simulink model "external_memory_test"  (R2020b)
settings: Solver=FixedStepDiscrete  StartTime=0.0  StopTime=80  RelTol=1e-3
InitFcn:
  | Feature_Width = 64;
  | Feature_Height = 64;
  | Weight_Width = 3;
  | Weight_Height = 3;
  | external_memory_test_init;
values from neighbouring files (symbols this model uses):
  Burst_Length = Feature_Weight_Length    [external_memory_test_init.m]
  byPass = 1    [external_memory_test_init.m]
  Conv_Padding = 0    [external_memory_test_init.m]
  Conv_Stride = 1    [external_memory_test_init.m]
  DDR_Depth = Weight_Length + Feature_Length + outFeature_Length    [external_memory_test_init.m]
  ddrInitData = single((rand(1,DDR_Depth)))    [external_memory_test_init.m]
  Duty_Cycle = 0.5    [external_memory_test_init.m]
  Feature_Area = Feature_Width * Feature_Height    [external_memory_test_init.m]
  Feature_Length = Phase_In * Feature_Area    [external_memory_test_init.m]
  inChannel = 3    [external_memory_test_init.m]
  outChannel = 2    [external_memory_test_init.m]
  outFeature_Length = outFeature_Width * outFeature_Height * Phase_Out    [external_memory_test_init.m]
  Pool_Stride = 2    [external_memory_test_init.m]
  Pool_Width = 2    [external_memory_test_init.m]
  Tc = 1    [external_memory_test_init.m]
  Ti = 1    [external_memory_test_init.m]
  To = 1    [external_memory_test_init.m]
  Tr = 1    [external_memory_test_init.m]
  Weight_Length = Phase_In * Weight_Area * Phase_Out    [external_memory_test_init.m]
undefined symbols (not defined in the file or in its folder): Conv_Step, Pool_Step, sigbuilder_block
libraries: hdlsllib x85, simulink x44, visionhdlutilities x16
(part 4 of 6)

== system external_memory_test/DUT/2DConvPE V1.3/Window Selector ==
  In1 : Inport
  valid : Inport  Port=2
  step : Inport  Port=3
  Add : Sum  Inputs=+-
  Compare To Zero : simulink/Logic and Bit Operations/Compare To Zero  relop===  OutDataTypeStr=boolean
  Constant : Constant  OutDataTypeStr=uint32
  Delay : Delay
  Delay1 : Delay  DelayLength=3
  Delay2 : Delay  DelayLength=1
  Delay3 : Delay  DelayLength=1
  Delay4 : Delay  DelayLength=1
  Logical Operator : Logic  Operator=NOT  AllPortsSameDT=off  OutDataTypeStr=boolean
  Logical Operator1 : Logic  Operator=OR  AllPortsSameDT=off  OutDataTypeStr=boolean
  Logical Operator2 : Logic  AllPortsSameDT=off  OutDataTypeStr=boolean
  Relational Operator : RelationalOperator  OutDataTypeStr=boolean  RndMeth=Nearest
  Selector1 : Selector  InputPortWidth=3  IndexOptions=Index vector (dialog)  Indices=[1]  OutputSizes=1
  Selector2 : Selector  InputPortWidth=3  IndexOptions=Index vector (dialog)  Indices=[2]  OutputSizes=1
  Selector3 : Selector  InputPortWidth=3  IndexOptions=Index vector (dialog)  Indices=[3]  OutputSizes=1
  Selector4 : Selector  InputPortWidth=3  IndexOptions=Index vector (dialog)  Indices=[1]  OutputSizes=1
  Selector5 : Selector  InputPortWidth=3  IndexOptions=Index vector (dialog)  Indices=[2]  OutputSizes=1
  Selector6 : Selector  InputPortWidth=3  IndexOptions=Index vector (dialog)  Indices=[3]  OutputSizes=1
  Selector7 : Selector  InputPortWidth=3  IndexOptions=Index vector (dialog)  Indices=[1]  OutputSizes=1
  Selector8 : Selector  InputPortWidth=3  IndexOptions=Index vector (dialog)  Indices=[2]  OutputSizes=1
  Selector9 : Selector  InputPortWidth=3  IndexOptions=Index vector (dialog)  Indices=[3]  OutputSizes=1
  Step Counter : hdlsllib/Sources/HDL Counter  CountType=Free running  CountInit=0  CountStep=1  CountMax=2^15  CountFromType=Initial value  CountFrom=0  CountResetPort=on  CountLoadPort=off  CountEnbPort=on  CountDirPort=off  CountDataType=Unsigned  CountWordLen=32  CountFracLen=0  CountSampTime=1
  Out1 : Outport
  Out2 : Outport  Port=2
  Out3 : Outport  Port=3
  Out4 : Outport  Port=4
  Out5 : Outport  Port=5
  Out6 : Outport  Port=6
  Out7 : Outport  Port=7
  Out8 : Outport  Port=8
  Out9 : Outport  Port=9
  Valid : Outport  Port=10
  wires:
  Selector2/1 -> Out2/1
  In1/1 -> Delay2/1, Delay1/1, Delay/1
  Selector1/1 -> Out1/1
  Selector3/1 -> Out3/1
  Selector8/1 -> Out5/1
  Selector9/1 -> Out6/1
  Selector7/1 -> Out4/1
  Delay/1 -> Selector9/1, Selector8/1, Selector7/1
  Selector5/1 -> Out8/1
  Selector6/1 -> Out9/1
  Selector4/1 -> Out7/1
  Delay1/1 -> Selector6/1, Selector5/1, Selector4/1
  Relational Operator/1 -> Logical Operator1/1
  Constant/1 -> Add/2
  Logical Operator2/1 -> Valid/1
  Compare To Zero/1 -> Logical Operator2/1
  Logical Operator1/1 -> Step Counter/1
  Logical Operator/1 -> Logical Operator1/2
  Delay4/1 -> Add/1
  Step Counter/1 -> Compare To Zero/1, Relational Operator/1
  Delay3/1 -> Logical Operator2/2, Step Counter/2, Logical Operator/1
  Add/1 -> Relational Operator/2
  Delay2/1 -> Selector3/1, Selector2/1, Selector1/1
  valid/1 -> Delay3/1
  step/1 -> Delay4/1

== system external_memory_test/DUT/DDR_Access/EdgeDetection2 ==
  In1 : Inport
  Delay : Delay  DelayLength=1
  Logical Operator : Logic  AllPortsSameDT=off  OutDataTypeStr=boolean
  Logical Operator1 : Logic  Operator=NOT  AllPortsSameDT=off  OutDataTypeStr=boolean
  Out1 : Outport  VectorParamsAs1DForOutWhenUnconnected=off
  wires:
  In1/1 -> Logical Operator/2, Delay/1
  Delay/1 -> Logical Operator1/1
  Logical Operator1/1 -> Logical Operator/1
  Logical Operator/1 -> Out1/1

== system external_memory_test/DUT/Input Buffer/Feature Buffer ==
  ram_wr_data : Inport
  ram_wr_addr : Inport  Port=2
  ram_wr_en : Inport  Port=3
  ram_rd_addr : Inport  Port=4
  Data Type Conversion : DataTypeConversion  OutDataTypeStr=uint16
  Data Type Conversion1 : DataTypeConversion  OutDataTypeStr=uint16
  Simple Dual Port RAM System : hdlsllib/HDL RAMs/Simple Dual Port RAM System  RAMType=Simple dual port  WriteOutputValue=New data  RAMInitialValue=0  SimulateUsing=Code generation
      settings: SourceProductName=HDL Coder
  ram_rd_data : Outport  VectorParamsAs1DForOutWhenUnconnected=off
  wires:
  Data Type Conversion/1 -> Simple Dual Port RAM System/2
  Data Type Conversion1/1 -> Simple Dual Port RAM System/4
  ram_wr_addr/1 -> Data Type Conversion/1
  Simple Dual Port RAM System/1 -> ram_rd_data/1
  ram_rd_addr/1 -> Data Type Conversion1/1
  ram_wr_en/1 -> Simple Dual Port RAM System/3
  ram_wr_data/1 -> Simple Dual Port RAM System/1

== system external_memory_test/DUT/Input Buffer/OutAddressLogic ==
  Weight_Length : Inport
  Weight_Area : Inport  Port=2
  Feature_Length : Inport  Port=3
  Feature_Area : Inport  Port=4
  Feature_Width : Inport  Port=5
  Feature_Height : Inport  Port=6
  outChannel : Inport  Port=7
  Out_enable : Inport  Port=8
  FeatureAddressOut : Subsystem
  Subsystem : Subsystem
  weight_ram_rd_addr : Outport
  featture_ram_rd_addr : Outport  Port=2
  feature_data_valid : Outport  Port=3
  weight_data_valid : Outport  Port=4
  PhaseOut_Count : Outport  Port=5
  wires:
  Feature_Length/1 -> FeatureAddressOut/1(Feature_Length)
  Out_enable/1 -> FeatureAddressOut/2(Out_Enable)
  Feature_Width/1 -> FeatureAddressOut/3(Feature_Width)
  FeatureAddressOut/1(count) -> featture_ram_rd_addr/1
  FeatureAddressOut/2(Out2) -> Subsystem/1(In1), feature_data_valid/1
  outChannel/1 -> FeatureAddressOut/4(outChannel)
  Feature_Area/1 -> Subsystem/2(Feature_Area)
  Weight_Length/1 -> Subsystem/3(Weight_Length)
  Weight_Area/1 -> Subsystem/4(Weight_Area)
  Subsystem/1(weight_ram_rd_addr) -> weight_ram_rd_addr/1
  Subsystem/2(valid) -> weight_data_valid/1
  Feature_Height/1 -> FeatureAddressOut/5(Feature_Height)
  FeatureAddressOut/3(PhaseOut_Count) -> PhaseOut_Count/1

== system external_memory_test/DUT/Input Buffer/SeparateWrite ==
  In1 : Inport
  In2 : Inport  Port=2
  Weight_Length : Inport  Port=3
  Compare To Zero : simulink/Logic and Bit Operations/Compare To Zero  relop=<  OutDataTypeStr=boolean
  Data Type Conversion : DataTypeConversion
  Logical Operator : Logic  Operator=NOT  AllPortsSameDT=off  OutDataTypeStr=boolean
  Logical Operator1 : Logic  AllPortsSameDT=off  OutDataTypeStr=boolean
  Logical Operator2 : Logic  AllPortsSameDT=off  OutDataTypeStr=boolean
  Minus : Sum  Inputs=+-
  Out1 : Outport
  Out2 : Outport  Port=2
  Out3 : Outport  Port=3
  wires:
  Logical Operator/1 -> Logical Operator2/2
  Minus/1 -> Data Type Conversion/1, Compare To Zero/1
  Logical Operator2/1 -> Out3/1
  Compare To Zero/1 -> Logical Operator/1, Logical Operator1/2
  In1/1 -> Logical Operator2/1, Logical Operator1/1
  In2/1 -> Minus/1
  Logical Operator1/1 -> Out1/1
  Weight_Length/1 -> Minus/2
  Data Type Conversion/1 -> Out2/1

== system external_memory_test/DUT/Input Buffer/Subsystem1 ==
  In1 : Inport
  Subsystem : Subsystem
  Terminator{,1..7} (8 alike) : Terminator
  Weight_Length : Outport
  Weight_Area : Outport  Port=2
  Feature_Length : Outport  Port=3
  Feature_Area : Outport  Port=4
  Feature_Width : Outport  Port=5
  Feature_Height : Outport  Port=6
  outChannel : Outport  Port=7
  wires:
  Subsystem/2(Weight_Area) -> Weight_Area/1
  Subsystem/12(outFeature_Height) -> Terminator5/1
  Subsystem/10(outFeature_Area) -> Terminator3/1
  Subsystem/13(Conv_Step) -> Terminator7/1
  Subsystem/9(outFeature_Length) -> Terminator2/1
  Subsystem/4(Weight_Height) -> Terminator1/1
  Subsystem/14(inChannel) -> Terminator6/1
  Subsystem/11(outFeature_Width) -> Terminator4/1
  Subsystem/3(Weight_Width) -> Terminator/1
  Subsystem/8(Feature_Height) -> Feature_Height/1
  Subsystem/1(Weight_Length) -> Weight_Length/1
  In1/1 -> Subsystem/1(In1)
  Subsystem/15(outChannel) -> outChannel/1
  Subsystem/5(Feature_Length) -> Feature_Length/1
  Subsystem/6(Feature_Area) -> Feature_Area/1
  Subsystem/7(Feature_Width) -> Feature_Width/1

== system external_memory_test/DUT/Input Buffer/Weight Buffer ==
  ram_wr_data : Inport
  ram_wr_addr : Inport  Port=2
  ram_wr_en : Inport  Port=3
  ram_rd_addr : Inport  Port=4
  Data Type Conversion : DataTypeConversion  OutDataTypeStr=uint16
  Data Type Conversion1 : DataTypeConversion  OutDataTypeStr=uint16
  Simple Dual Port RAM System : hdlsllib/HDL RAMs/Simple Dual Port RAM System  RAMType=Simple dual port  WriteOutputValue=New data  RAMInitialValue=0  SimulateUsing=Code generation
      settings: SourceProductName=HDL Coder
  ram_rd_data : Outport  VectorParamsAs1DForOutWhenUnconnected=off
  wires:
  Data Type Conversion/1 -> Simple Dual Port RAM System/2
  Data Type Conversion1/1 -> Simple Dual Port RAM System/4
  ram_wr_addr/1 -> Data Type Conversion/1
  Simple Dual Port RAM System/1 -> ram_rd_data/1
  ram_rd_addr/1 -> Data Type Conversion1/1
  ram_wr_en/1 -> Simple Dual Port RAM System/3
  ram_wr_data/1 -> Simple Dual Port RAM System/1

== system external_memory_test/DUT/outBuffer/Out Buffer ==
  ram_wr_data : Inport
  ram_wr_addr : Inport  Port=2
  ram_wr_en : Inport  Port=3
  ram_rd_addr : Inport  Port=4
  Cast : DataTypeConversion  OutDataTypeStr=uint32
  Data Type Conversion : DataTypeConversion  OutDataTypeStr=uint16
  Data Type Conversion1 : DataTypeConversion  OutDataTypeStr=uint16
  Simple Dual Port RAM System : hdlsllib/HDL RAMs/Simple Dual Port RAM System  RAMType=Simple dual port  WriteOutputValue=New data  RAMInitialValue=0  SimulateUsing=Code generation
      settings: SourceProductName=HDL Coder
  ram_rd_data : Outport  VectorParamsAs1DForOutWhenUnconnected=off
  wires:
  Data Type Conversion/1 -> Simple Dual Port RAM System/2
  Data Type Conversion1/1 -> Simple Dual Port RAM System/4
  ram_wr_addr/1 -> Data Type Conversion/1
  Simple Dual Port RAM System/1 -> Cast/1
  ram_rd_addr/1 -> Data Type Conversion1/1
  ram_wr_en/1 -> Simple Dual Port RAM System/3
  ram_wr_data/1 -> Simple Dual Port RAM System/1
  Cast/1 -> ram_rd_data/1

== system external_memory_test/InputSubsystem/Subsystem1/Signal Builder-Simulation ==
  Demux : Demux  Tag=STV Demux  Outputs=3
      settings: DisplayOption=none
  FromWs : FromWorkspace  Tag=STV FromWs  VariableName=tuvar  SampleTime=0.001  ZeroCross=off  OutputAfterFinalValue=Holding final value
      SigBuilderData=|
      | common.afterFinalStr = 'Hold final value'
      | common.sampleTime = '0.001'
      | dataSet.timeRange = [0 80]
      | dataSet.name = 'Group 1'
      | sbobj.Groups.Name = 'Group 1'
      | sbobj.Groups.Signals(1).Name = 'start'
      | sbobj.Groups.Signals(1).XData = [0 29 29 30 30 60 60 61 61 80]
      | sbobj.Groups.Signals(1).YData = [0 0 1 1 0 0 1 1 0 0]
      | sbobj.Groups.Signals(2).Name = 'from_ddr_to_ram'
      | sbobj.Groups.Signals(2).XData = [0 58.6 58.6 80]
      | sbobj.Groups.Signals(2).YData = [1 1 0 0]
      | sbobj.Groups.Signals(3).Name = 'conv_en'
      | sbobj.Groups.Signals(3).XData = [0 31.3 31.3 50 80]
      | sbobj.Groups.Signals(3).YData = [0 0 1 0.99 0.99]
      | sbobj.Groups.TimeRange = [0 80]
  start : Outport  Tag=STV Outport  VectorParamsAs1DForOutWhenUnconnected=off
  from_ddr_to_ram : Outport  Tag=STV Outport  Port=2  VectorParamsAs1DForOutWhenUnconnected=off
  conv_en : Outport  Tag=STV Outport  Port=3
  wires:
  Demux/1 -> start/1
  Demux/2 -> from_ddr_to_ram/1
  Demux/3 -> conv_en/1
  FromWs/1 -> Demux/1

== system external_memory_test/OutputSubsystem/to_MATLAB/to Matlab ==
  In1 : Inport
  Enable : EnablePort
  To Workspace : ToWorkspace  VariableName=DDR_WR_DATA  SampleTime=-1
  wires:
  In1/1 -> To Workspace/1

== system external_memory_test/DDR/wrLogic/Wr_control/AckGen ==
  axiWrLen : Inport
  wrEnb : Inport  Port=2
  ddr_wr_rdy : Inport  Port=3
  Delay : Delay  DelayLength=1
  Delay1 : Delay  DelayLength=1
  ValwrLenCnt : hdlsllib/Sources/HDL Counter  CountType=Free running  CountInit=0  CountStep=1  CountMax=DDR3_DEPTH  CountFromType=Initial value  CountFrom=0  CountResetPort=on  CountLoadPort=off  CountEnbPort=on  CountDirPort=off  CountDataType=Unsigned  CountWordLen=32  CountFracLen=0  CountSampTime=1
  axiWrLen!=0 : simulink/Logic and Bit Operations/Compare To Constant  relop=~=  const=0  OutDataTypeStr=boolean
  "axiWrLen-1==cnt & axiWrLen!=0 " : Logic  Inputs=3  IconShape=distinctive  AllPortsSameDT=off  OutDataTypeStr=boolean
  axiWrLen==cnt+1 : RelationalOperator  Operator===  OutDataTypeStr=boolean  RndMeth=Nearest
  edgeDet : Subsystem
  if cnt < axiWrLen : RelationalOperator  Operator=<=  OutDataTypeStr=boolean  RndMeth=Nearest
  ram_wr_enb cond : Logic  IconShape=distinctive  AllPortsSameDT=off  OutDataTypeStr=boolean
  ram_wr_enb cond1 : Logic  IconShape=distinctive  AllPortsSameDT=off  OutDataTypeStr=boolean
  ack : Outport  VectorParamsAs1DForOutWhenUnconnected=off
  ValAddEnb : Outport  Port=2  VectorParamsAs1DForOutWhenUnconnected=off
  ram_addr : Outport  Port=3  VectorParamsAs1DForOutWhenUnconnected=off
  wires:
  "axiWrLen-1==cnt & axiWrLen!=0 "/1 -> edgeDet/1(ackIn)
  edgeDet/1(ackOut) -> ack/1, Delay/1
  axiWrLen==cnt+1/1 -> "axiWrLen-1==cnt & axiWrLen!=0 "/2
  axiWrLen!=0/1 -> "axiWrLen-1==cnt & axiWrLen!=0 "/3
  wrEnb/1 -> ram_wr_enb cond/1
  if cnt < axiWrLen/1 -> ram_wr_enb cond1/2
  axiWrLen/1 -> axiWrLen==cnt+1/2, axiWrLen!=0/1, if cnt < axiWrLen/2
  ValwrLenCnt/1 -> axiWrLen==cnt+1/1, if cnt < axiWrLen/1, ram_addr/1
  ddr_wr_rdy/1 -> ram_wr_enb cond/2
  ram_wr_enb cond/1 -> ram_wr_enb cond1/1, Delay1/1, ValwrLenCnt/2
  ram_wr_enb cond1/1 -> ValAddEnb/1
  Delay/1 -> ValwrLenCnt/1
  Delay1/1 -> "axiWrLen-1==cnt & axiWrLen!=0 "/1

== system external_memory_test/DUT/2DConvPE V1.0/Address Logic/  ==
  In1 : Inport
  In2 : Inport  Port=2
  Constant1 : Constant  Value=0  OutDataTypeStr=uint32
  Constant2 : Constant  Value=0  OutDataTypeStr=uint32
  Logical Operator3 : Logic  Operator=NOT  AllPortsSameDT=off  OutDataTypeStr=boolean
  Switch : Switch  Criteria=u2 ~= 0
  Switch1 : Switch  Criteria=u2 ~= 0
  addr_bit_sel1 : hdlsllib/Logic and Bit Operations/Bit Slice  lidx=12  ridx=0
  addr_bit_sel2 : hdlsllib/Logic and Bit Operations/Bit Slice  lidx=12  ridx=0
  W : Outport
  R : Outport  Port=2
  wires:
  In2/1 -> Switch/2, Logical Operator3/1
  Constant1/1 -> Switch/1
  Switch1/1 -> addr_bit_sel1/1
  In1/1 -> Switch1/3, Switch/3
  Logical Operator3/1 -> Switch1/2
  Constant2/1 -> Switch1/1
  Switch/1 -> addr_bit_sel2/1
  addr_bit_sel1/1 -> W/1  "vec_wr_addr"
  addr_bit_sel2/1 -> R/1  "vec_wr_addr"

== system external_memory_test/DUT/2DConvPE V1.0/LIne Buffer/Line Buffer ==
  Stream_In : Inport
  Stream_Valid : Inport  Port=2
  Feature_Area : Inport  Port=3
  Feature_Width : Inport  Port=4
  CtrlGen : Subsystem
  Line Buffer : visionhdlutilities/Line Buffer  NeighborhoodSize=[3 1]  PaddingMethod=Constant  PaddingValue=0  LineBufferSize=128  SimulateUsing=Code generation
      settings: SourceProductBaseCode=VT
  pixel : Outport
  ctrl : Outport  Port=2
  shftEnable : Outport  Port=3
  wires:
  Feature_Area/1 -> CtrlGen/3(Feature_Area)
  Line Buffer/2 -> ctrl/1
  CtrlGen/1(StreamOut) -> Line Buffer/1
  Feature_Width/1 -> CtrlGen/4(Feature_Width)
  Stream_In/1 -> CtrlGen/1(Stream_In)
  CtrlGen/2(Ctrl) -> Line Buffer/2
  Stream_Valid/1 -> CtrlGen/2(Stream_Valid)
  Line Buffer/3 -> shftEnable/1
  Line Buffer/1 -> pixel/1

== system external_memory_test/DUT/2DConvPE V1.0/LIne Buffer/OutValidGen ==
  In1 : Inport
  Weight_Width : Inport  Port=2
  Feature_Height : Inport  Port=3
  Compare To Constant : simulink/Logic and Bit Operations/Compare To Constant  relop=>  const=0  OutDataTypeStr=boolean
  Constant : Constant  OutDataTypeStr=uint32  SampleTime=-1
  Delay2 : Delay  DelayLength=1
  Logical Operator1 : Logic  Operator=NOT  AllPortsSameDT=off  OutDataTypeStr=boolean
  Logical Operator2 : Logic  Operator=OR  AllPortsSameDT=off  OutDataTypeStr=boolean
  Logical Operator3 : Logic  Inputs=4  AllPortsSameDT=off  OutDataTypeStr=boolean
  Logical Operator4 : Logic  Operator=NOT  AllPortsSameDT=off  OutDataTypeStr=boolean
  Logical Operator5 : Logic  Operator=OR  AllPortsSameDT=off  OutDataTypeStr=boolean
  Logical Operator6 : Logic  Operator=NOT  Inputs=3  AllPortsSameDT=off  OutDataTypeStr=boolean
  Minus1 : Sum  Inputs=+--
  Minus2 : Sum  Inputs=+-
  NumRow_Counter : hdlsllib/Sources/HDL Counter  CountType=Free running  CountInit=0  CountStep=1  CountMax=2^15  CountFromType=Initial value  CountFrom=0  CountResetPort=on  CountLoadPort=off  CountEnbPort=on  CountDirPort=off  CountDataType=Unsigned  CountWordLen=32  CountFracLen=0  CountSampTime=1
  Pixel Control Bus Selector : BusSelector  OutputSignals=hStart,hEnd,vStart,vEnd,valid
  Relational Operator1 : RelationalOperator  Operator=<  OutDataTypeStr=boolean  RndMeth=Nearest
  Relational Operator2 : RelationalOperator  Operator=<=  OutDataTypeStr=boolean  RndMeth=Nearest
  Row_Counter : hdlsllib/Sources/HDL Counter  CountType=Free running  CountInit=0  CountStep=1  CountMax=2^15  CountFromType=Initial value  CountFrom=0  CountResetPort=on  CountLoadPort=off  CountEnbPort=on  CountDirPort=off  CountDataType=Unsigned  CountWordLen=32  CountFracLen=0  CountSampTime=1
  Terminator1 : Terminator
  valid : Outport
  wires:
  Compare To Constant/1 -> Logical Operator3/2
  NumRow_Counter/1 -> Relational Operator2/2, Compare To Constant/1
  Pixel Control Bus Selector/1 -> NumRow_Counter/2, Logical Operator2/1  "<hStart>"
  Minus2/1 -> Relational Operator2/1
  Relational Operator1/1 -> Logical Operator4/1
  Logical Operator1/1 -> Logical Operator2/2
  Pixel Control Bus Selector/3 -> Logical Operator5/1  "<vStart>"
  Feature_Height/1 -> Minus2/1
  Minus1/1 -> Relational Operator1/2
  Row_Counter/1 -> Relational Operator1/1
  Pixel Control Bus Selector/5 -> Logical Operator1/1, Row_Counter/2, Logical Operator3/3  "<valid>"
  Weight_Width/1 -> Minus1/1
  Pixel Control Bus Selector/2 -> Terminator1/1  "<hEnd>"
  Delay2/1 -> Pixel Control Bus Selector/1
  Constant/1 -> Minus1/3, Minus1/2, Minus2/2
  Logical Operator6/1 -> Logical Operator3/1
  Logical Operator5/1 -> NumRow_Counter/1
  Pixel Control Bus Selector/4 -> Logical Operator5/2  "<vEnd>"
  Relational Operator2/1 -> Logical Operator6/1
  Logical Operator2/1 -> Row_Counter/1
  Logical Operator4/1 -> Logical Operator3/4
  Logical Operator3/1 -> valid/1
  In1/1 -> Delay2/1

== system external_memory_test/DUT/2DConvPE V1.0/MaxPooling/Comparator ==
  In1 : Inport
  In2 : Inport  Port=2
  In3 : Inport  Port=3
  In4 : Inport  Port=4
  Valid : Inport  Port=5
  Delay{,1..4} (5 alike) : Delay  DelayLength=1
  Relational Operator : RelationalOperator  Operator=>  OutDataTypeStr=boolean  RndMeth=Nearest
  Relational Operator1 : RelationalOperator  Operator=>  OutDataTypeStr=boolean  RndMeth=Nearest
  Relational Operator2 : RelationalOperator  Operator=>  OutDataTypeStr=boolean  RndMeth=Nearest
  Switch : Switch  Criteria=u2 > Threshold
  Switch1 : Switch  Criteria=u2 > Threshold
  Switch2 : Switch  Criteria=u2 > Threshold
  Out1 : Outport
  outvalid : Outport  Port=2
  wires:
  Switch1/1 -> Relational Operator2/2, Switch2/3
  Switch/1 -> Switch2/1, Relational Operator2/1
  Delay/1 -> Switch/1, Relational Operator/1
  Relational Operator/1 -> Switch/2
  Relational Operator1/1 -> Switch1/2
  In2/1 -> Delay1/1
  In3/1 -> Delay2/1
  Relational Operator2/1 -> Switch2/2
  In4/1 -> Delay3/1
  Switch2/1 -> Out1/1
  Valid/1 -> Delay4/1
  Delay1/1 -> Relational Operator/2, Switch/3
  Delay2/1 -> Switch1/1, Relational Operator1/1
  In1/1 -> Delay/1
  Delay3/1 -> Relational Operator1/2, Switch1/3
  Delay4/1 -> outvalid/1

== system external_memory_test/DUT/2DConvPE V1.0/MaxPooling/Line Buffer1 ==
  Stream_In : Inport
  Stream_Valid : Inport  Port=2
  Feature_Area : Inport  Port=3
  Feature_Width : Inport  Port=4
  CtrlGen : Subsystem
  Line Buffer : visionhdlutilities/Line Buffer  NeighborhoodSize=[2 1]  PaddingMethod=Constant  PaddingValue=0  LineBufferSize=128  SimulateUsing=Code generation
      settings: SourceProductBaseCode=VT
  pixel : Outport
  ctrl : Outport  Port=2
  shftEnable : Outport  Port=3
  wires:
  Feature_Area/1 -> CtrlGen/3(Feature_Area)
  Line Buffer/2 -> ctrl/1
  CtrlGen/1(StreamOut) -> Line Buffer/1
  Feature_Width/1 -> CtrlGen/4(Feature_Width)
  Stream_In/1 -> CtrlGen/1(Stream_In)
  CtrlGen/2(Ctrl) -> Line Buffer/2
  Stream_Valid/1 -> CtrlGen/2(Stream_Valid)
  Line Buffer/3 -> shftEnable/1
  Line Buffer/1 -> pixel/1

== system external_memory_test/DUT/2DConvPE V1.0/MaxPooling/OutValidGen ==
  ctrl : Inport
  Window_Width : Inport  Port=2
  Feature_Height : Inport  Port=3
  Compare To Constant : simulink/Logic and Bit Operations/Compare To Constant  Commented=on  relop=>  const=0  OutDataTypeStr=boolean
  Constant : Constant  OutDataTypeStr=uint32  SampleTime=-1
  Delay36 : Delay  DelayLength=1
  Logical Operator1 : Logic  Operator=NOT  AllPortsSameDT=off  OutDataTypeStr=boolean
  Logical Operator3 : Logic  Inputs=3  AllPortsSameDT=off  OutDataTypeStr=boolean
  Logical Operator4 : Logic  Operator=NOT  AllPortsSameDT=off  OutDataTypeStr=boolean
  Logical Operator5 : Logic  Operator=OR  AllPortsSameDT=off  OutDataTypeStr=boolean
  Logical Operator6 : Logic  Operator=NOT  Inputs=3  AllPortsSameDT=off  OutDataTypeStr=boolean
  Minus1 : Sum  Inputs=+-
  Minus2 : Sum  Inputs=+-
  NumRow_Counter : hdlsllib/Sources/HDL Counter  CountType=Free running  CountInit=0  CountStep=1  CountMax=2^15  CountFromType=Initial value  CountFrom=0  CountResetPort=on  CountLoadPort=off  CountEnbPort=on  CountDirPort=off  CountDataType=Unsigned  CountWordLen=32  CountFracLen=0  CountSampTime=1
  Pixel Control Bus Selector : BusSelector  OutputSignals=hStart,hEnd,vStart,vEnd,valid
  Relational Operator1 : RelationalOperator  Operator=<  OutDataTypeStr=boolean  RndMeth=Nearest
  Relational Operator2 : RelationalOperator  Operator=<=  OutDataTypeStr=boolean  RndMeth=Nearest
  Row_Counter : hdlsllib/Sources/HDL Counter  CountType=Free running  CountInit=0  CountStep=1  CountMax=2^15  CountFromType=Initial value  CountFrom=0  CountResetPort=on  CountLoadPort=off  CountEnbPort=on  CountDirPort=off  CountDataType=Unsigned  CountWordLen=32  CountFracLen=0  CountSampTime=1
  Terminator1 : Terminator
  Out1 : Outport
  wires:
  Compare To Constant/1 -> ?
  NumRow_Counter/1 -> Relational Operator2/2, Compare To Constant/1
  Pixel Control Bus Selector/1 -> NumRow_Counter/2  "<hStart>"
  Minus2/1 -> Relational Operator2/1
  Relational Operator1/1 -> Logical Operator4/1
  Pixel Control Bus Selector/3 -> Logical Operator5/1  "<vStart>"
  Feature_Height/1 -> Minus2/1
  Minus1/1 -> Relational Operator1/2
  Row_Counter/1 -> Relational Operator1/1
  Pixel Control Bus Selector/5 -> Row_Counter/2, Logical Operator1/1, Logical Operator3/2  "<valid>"
  Window_Width/1 -> Minus1/1
  Pixel Control Bus Selector/2 -> Terminator1/1  "<hEnd>"
  Delay36/1 -> Pixel Control Bus Selector/1
  Constant/1 -> Minus1/2, Minus2/2
  Logical Operator6/1 -> Logical Operator3/1
  Logical Operator5/1 -> NumRow_Counter/1
  Pixel Control Bus Selector/4 -> Logical Operator5/2  "<vEnd>"
  Relational Operator2/1 -> Logical Operator6/1
  Logical Operator1/1 -> Row_Counter/1
  Logical Operator4/1 -> Logical Operator3/3
  Logical Operator3/1 -> Out1/1
  ctrl/1 -> Delay36/1

== system external_memory_test/DUT/2DConvPE V1.0/MaxPooling/window Selector ==
  pixel : Inport
  valid : Inport  Port=2
  step : Inport  Port=3
  Add : Sum  Inputs=+-
  Compare To Zero : simulink/Logic and Bit Operations/Compare To Zero  relop===  OutDataTypeStr=boolean
  Constant : Constant  OutDataTypeStr=uint32
  Delay : Delay
  Delay1 : Delay  DelayLength=1
  Delay36 : Delay  DelayLength=1
  Logical Operator : Logic  Operator=NOT  AllPortsSameDT=off  OutDataTypeStr=boolean
  Logical Operator1 : Logic  Operator=OR  AllPortsSameDT=off  OutDataTypeStr=boolean
  Logical Operator2 : Logic  AllPortsSameDT=off  OutDataTypeStr=boolean
  Relational Operator : RelationalOperator  OutDataTypeStr=boolean  RndMeth=Nearest
  Selector1 : Selector  InputPortWidth=2  IndexOptions=Index vector (dialog)  Indices=[1]  OutputSizes=1
  Selector2 : Selector  InputPortWidth=2  IndexOptions=Index vector (dialog)  Indices=[2]  OutputSizes=1
  Selector3 : Selector  InputPortWidth=2  IndexOptions=Index vector (dialog)  Indices=[1]  OutputSizes=1
  Selector4 : Selector  InputPortWidth=2  IndexOptions=Index vector (dialog)  Indices=[2]  OutputSizes=1
  Step Counter : hdlsllib/Sources/HDL Counter  CountType=Free running  CountInit=0  CountStep=1  CountMax=2^15  CountFromType=Initial value  CountFrom=0  CountResetPort=on  CountLoadPort=off  CountEnbPort=on  CountDirPort=off  CountDataType=Unsigned  CountWordLen=32  CountFracLen=0  CountSampTime=1
  Out1 : Outport
  Out2 : Outport  Port=2
  Out3 : Outport  Port=3
  Out4 : Outport  Port=4
  Valid : Outport  Port=5
  wires:
  Selector2/1 -> Out2/1
  Delay/1 -> Selector4/1, Selector3/1
  Selector3/1 -> Out3/1
  Selector1/1 -> Out1/1
  Selector4/1 -> Out4/1
  pixel/1 -> Delay36/1, Delay/1
  Step Counter/1 -> Compare To Zero/1, Relational Operator/1
  Delay1/1 -> Logical Operator2/2, Step Counter/2, Logical Operator/1
  Logical Operator/1 -> Logical Operator1/2
  step/1 -> Add/1
  Constant/1 -> Add/2
  Add/1 -> Relational Operator/2
  Relational Operator/1 -> Logical Operator1/1
  Logical Operator1/1 -> Step Counter/1
  Compare To Zero/1 -> Logical Operator2/1
  Logical Operator2/1 -> Valid/1
  Delay36/1 -> Selector2/1, Selector1/1
  valid/1 -> Delay1/1

== system external_memory_test/DUT/2DConvPE V1.1/Address Logic/  ==
  In1 : Inport
  In2 : Inport  Port=2
  Constant1 : Constant  Value=0  OutDataTypeStr=uint32
  Constant2 : Constant  Value=0  OutDataTypeStr=uint32
  Logical Operator3 : Logic  Operator=NOT  AllPortsSameDT=off  OutDataTypeStr=boolean
  Switch : Switch  Criteria=u2 ~= 0
  Switch1 : Switch  Criteria=u2 ~= 0
  addr_bit_sel1 : hdlsllib/Logic and Bit Operations/Bit Slice  lidx=12  ridx=0
  addr_bit_sel2 : hdlsllib/Logic and Bit Operations/Bit Slice  lidx=12  ridx=0
  W : Outport
  R : Outport  Port=2
  wires:
  In2/1 -> Switch/2, Logical Operator3/1
  Constant1/1 -> Switch/1
  Switch1/1 -> addr_bit_sel1/1
  In1/1 -> Switch1/3, Switch/3
  Logical Operator3/1 -> Switch1/2
  Constant2/1 -> Switch1/1
  Switch/1 -> addr_bit_sel2/1
  addr_bit_sel1/1 -> W/1  "vec_wr_addr"
  addr_bit_sel2/1 -> R/1  "vec_wr_addr"

== system external_memory_test/DUT/2DConvPE V1.1/LIne Buffer/Line Buffer ==
  Stream_In : Inport
  Stream_Valid : Inport  Port=2
  Feature_Area : Inport  Port=3
  Feature_Width : Inport  Port=4
  CtrlGen : Subsystem
  Line Buffer : visionhdlutilities/Line Buffer  NeighborhoodSize=[3 1]  PaddingMethod=Constant  PaddingValue=0  LineBufferSize=128  SimulateUsing=Code generation
      settings: SourceProductBaseCode=VT
  pixel : Outport
  ctrl : Outport  Port=2
  shftEnable : Outport  Port=3
  wires:
  Feature_Area/1 -> CtrlGen/3(Feature_Area)
  Line Buffer/2 -> ctrl/1
  CtrlGen/1(StreamOut) -> Line Buffer/1
  Feature_Width/1 -> CtrlGen/4(Feature_Width)
  Stream_In/1 -> CtrlGen/1(Stream_In)
  CtrlGen/2(Ctrl) -> Line Buffer/2
  Stream_Valid/1 -> CtrlGen/2(Stream_Valid)
  Line Buffer/3 -> shftEnable/1
  Line Buffer/1 -> pixel/1

== system external_memory_test/DUT/2DConvPE V1.1/LIne Buffer/OutValidGen ==
  In1 : Inport
  Weight_Width : Inport  Port=2
  Feature_Height : Inport  Port=3
  Compare To Constant : simulink/Logic and Bit Operations/Compare To Constant  relop=>  const=0  OutDataTypeStr=boolean
  Constant : Constant  OutDataTypeStr=uint32  SampleTime=-1
  Delay2 : Delay  DelayLength=1
  Logical Operator1 : Logic  Operator=NOT  AllPortsSameDT=off  OutDataTypeStr=boolean
  Logical Operator2 : Logic  Operator=OR  AllPortsSameDT=off  OutDataTypeStr=boolean
  Logical Operator3 : Logic  Inputs=4  AllPortsSameDT=off  OutDataTypeStr=boolean
  Logical Operator4 : Logic  Operator=NOT  AllPortsSameDT=off  OutDataTypeStr=boolean
  Logical Operator5 : Logic  Operator=OR  AllPortsSameDT=off  OutDataTypeStr=boolean
  Logical Operator6 : Logic  Operator=NOT  Inputs=3  AllPortsSameDT=off  OutDataTypeStr=boolean
  Minus1 : Sum  Inputs=+--
  Minus2 : Sum  Inputs=+-
  NumRow_Counter : hdlsllib/Sources/HDL Counter  CountType=Free running  CountInit=0  CountStep=1  CountMax=2^15  CountFromType=Initial value  CountFrom=0  CountResetPort=on  CountLoadPort=off  CountEnbPort=on  CountDirPort=off  CountDataType=Unsigned  CountWordLen=32  CountFracLen=0  CountSampTime=1
  Pixel Control Bus Selector : BusSelector  OutputSignals=hStart,hEnd,vStart,vEnd,valid
  Relational Operator1 : RelationalOperator  Operator=<  OutDataTypeStr=boolean  RndMeth=Nearest
  Relational Operator2 : RelationalOperator  Operator=<=  OutDataTypeStr=boolean  RndMeth=Nearest
  Row_Counter : hdlsllib/Sources/HDL Counter  CountType=Free running  CountInit=0  CountStep=1  CountMax=2^15  CountFromType=Initial value  CountFrom=0  CountResetPort=on  CountLoadPort=off  CountEnbPort=on  CountDirPort=off  CountDataType=Unsigned  CountWordLen=32  CountFracLen=0  CountSampTime=1
  Terminator1 : Terminator
  valid : Outport
  wires:
  Compare To Constant/1 -> Logical Operator3/2
  NumRow_Counter/1 -> Relational Operator2/2, Compare To Constant/1
  Pixel Control Bus Selector/1 -> NumRow_Counter/2, Logical Operator2/1  "<hStart>"
  Minus2/1 -> Relational Operator2/1
  Relational Operator1/1 -> Logical Operator4/1
  Logical Operator1/1 -> Logical Operator2/2
  Pixel Control Bus Selector/3 -> Logical Operator5/1  "<vStart>"
  Feature_Height/1 -> Minus2/1
  Minus1/1 -> Relational Operator1/2
  Row_Counter/1 -> Relational Operator1/1
  Pixel Control Bus Selector/5 -> Logical Operator1/1, Row_Counter/2, Logical Operator3/3  "<valid>"
  Weight_Width/1 -> Minus1/1
  Pixel Control Bus Selector/2 -> Terminator1/1  "<hEnd>"
  Delay2/1 -> Pixel Control Bus Selector/1
  Constant/1 -> Minus1/3, Minus1/2, Minus2/2
  Logical Operator6/1 -> Logical Operator3/1
  Logical Operator5/1 -> NumRow_Counter/1
  Pixel Control Bus Selector/4 -> Logical Operator5/2  "<vEnd>"
  Relational Operator2/1 -> Logical Operator6/1
  Logical Operator2/1 -> Row_Counter/1
  Logical Operator4/1 -> Logical Operator3/4
  Logical Operator3/1 -> valid/1
  In1/1 -> Delay2/1

== system external_memory_test/DUT/2DConvPE V1.1/MaxPooling/Comparator ==
  In1 : Inport
  In2 : Inport  Port=2
  In3 : Inport  Port=3
  In4 : Inport  Port=4
  Valid : Inport  Port=5
  Delay{,1..4} (5 alike) : Delay  DelayLength=1
  Relational Operator : RelationalOperator  Operator=>  OutDataTypeStr=boolean  RndMeth=Nearest
  Relational Operator1 : RelationalOperator  Operator=>  OutDataTypeStr=boolean  RndMeth=Nearest
  Relational Operator2 : RelationalOperator  Operator=>  OutDataTypeStr=boolean  RndMeth=Nearest
  Switch : Switch  Criteria=u2 > Threshold
  Switch1 : Switch  Criteria=u2 > Threshold
  Switch2 : Switch  Criteria=u2 > Threshold
  Out1 : Outport
  outvalid : Outport  Port=2
  wires:
  Switch1/1 -> Relational Operator2/2, Switch2/3
  Switch/1 -> Switch2/1, Relational Operator2/1
  Delay/1 -> Switch/1, Relational Operator/1
  Relational Operator/1 -> Switch/2
  Relational Operator1/1 -> Switch1/2
  In2/1 -> Delay1/1
  In3/1 -> Delay2/1
  Relational Operator2/1 -> Switch2/2
  In4/1 -> Delay3/1
  Switch2/1 -> Out1/1
  Valid/1 -> Delay4/1
  Delay1/1 -> Relational Operator/2, Switch/3
  Delay2/1 -> Switch1/1, Relational Operator1/1
  In1/1 -> Delay/1
  Delay3/1 -> Relational Operator1/2, Switch1/3
  Delay4/1 -> outvalid/1

== system external_memory_test/DUT/2DConvPE V1.1/MaxPooling/Line Buffer1 ==
  Stream_In : Inport
  Stream_Valid : Inport  Port=2
  Feature_Area : Inport  Port=3
  Feature_Width : Inport  Port=4
  CtrlGen : Subsystem
  Line Buffer : visionhdlutilities/Line Buffer  NeighborhoodSize=[2 1]  PaddingMethod=Constant  PaddingValue=0  LineBufferSize=128  SimulateUsing=Code generation
      settings: SourceProductBaseCode=VT
  pixel : Outport
  ctrl : Outport  Port=2
  shftEnable : Outport  Port=3
  wires:
  Feature_Area/1 -> CtrlGen/3(Feature_Area)
  Line Buffer/2 -> ctrl/1
  CtrlGen/1(StreamOut) -> Line Buffer/1
  Feature_Width/1 -> CtrlGen/4(Feature_Width)
  Stream_In/1 -> CtrlGen/1(Stream_In)
  CtrlGen/2(Ctrl) -> Line Buffer/2
  Stream_Valid/1 -> CtrlGen/2(Stream_Valid)
  Line Buffer/3 -> shftEnable/1
  Line Buffer/1 -> pixel/1

== system external_memory_test/DUT/2DConvPE V1.1/MaxPooling/OutValidGen ==
  ctrl : Inport
  Window_Width : Inport  Port=2
  Feature_Height : Inport  Port=3
  Compare To Constant : simulink/Logic and Bit Operations/Compare To Constant  Commented=on  relop=>  const=0  OutDataTypeStr=boolean
  Constant : Constant  OutDataTypeStr=uint32  SampleTime=-1
  Delay36 : Delay  DelayLength=1
  Logical Operator1 : Logic  Operator=NOT  AllPortsSameDT=off  OutDataTypeStr=boolean
  Logical Operator3 : Logic  Inputs=3  AllPortsSameDT=off  OutDataTypeStr=boolean
  Logical Operator4 : Logic  Operator=NOT  AllPortsSameDT=off  OutDataTypeStr=boolean
  Logical Operator5 : Logic  Operator=OR  AllPortsSameDT=off  OutDataTypeStr=boolean
  Logical Operator6 : Logic  Operator=NOT  Inputs=3  AllPortsSameDT=off  OutDataTypeStr=boolean
  Minus1 : Sum  Inputs=+-
  Minus2 : Sum  Inputs=+-
  NumRow_Counter : hdlsllib/Sources/HDL Counter  CountType=Free running  CountInit=0  CountStep=1  CountMax=2^15  CountFromType=Initial value  CountFrom=0  CountResetPort=on  CountLoadPort=off  CountEnbPort=on  CountDirPort=off  CountDataType=Unsigned  CountWordLen=32  CountFracLen=0  CountSampTime=1
  Pixel Control Bus Selector : BusSelector  OutputSignals=hStart,hEnd,vStart,vEnd,valid
  Relational Operator1 : RelationalOperator  Operator=<  OutDataTypeStr=boolean  RndMeth=Nearest
  Relational Operator2 : RelationalOperator  Operator=<=  OutDataTypeStr=boolean  RndMeth=Nearest
  Row_Counter : hdlsllib/Sources/HDL Counter  CountType=Free running  CountInit=0  CountStep=1  CountMax=2^15  CountFromType=Initial value  CountFrom=0  CountResetPort=on  CountLoadPort=off  CountEnbPort=on  CountDirPort=off  CountDataType=Unsigned  CountWordLen=32  CountFracLen=0  CountSampTime=1
  Terminator1 : Terminator
  Out1 : Outport
  wires:
  NumRow_Counter/1 -> Relational Operator2/2, Compare To Constant/1
  Pixel Control Bus Selector/1 -> NumRow_Counter/2  "<hStart>"
  Minus2/1 -> Relational Operator2/1
  Relational Operator1/1 -> Logical Operator4/1
  Pixel Control Bus Selector/3 -> Logical Operator5/1  "<vStart>"
  Feature_Height/1 -> Minus2/1
  Minus1/1 -> Relational Operator1/2
  Row_Counter/1 -> Relational Operator1/1
  Pixel Control Bus Selector/5 -> Row_Counter/2, Logical Operator1/1, Logical Operator3/2  "<valid>"
  Window_Width/1 -> Minus1/1
  Pixel Control Bus Selector/2 -> Terminator1/1  "<hEnd>"
  Delay36/1 -> Pixel Control Bus Selector/1
  Constant/1 -> Minus1/2, Minus2/2
  Logical Operator6/1 -> Logical Operator3/1
  Logical Operator5/1 -> NumRow_Counter/1
  Pixel Control Bus Selector/4 -> Logical Operator5/2  "<vEnd>"
  Relational Operator2/1 -> Logical Operator6/1
  Logical Operator1/1 -> Row_Counter/1
  Logical Operator4/1 -> Logical Operator3/3
  Logical Operator3/1 -> Out1/1
  ctrl/1 -> Delay36/1

== system external_memory_test/DUT/2DConvPE V1.1/MaxPooling/window Selector ==
  pixel : Inport
  valid : Inport  Port=2
  step : Inport  Port=3
  Add : Sum  Inputs=+-
  Compare To Zero : simulink/Logic and Bit Operations/Compare To Zero  relop===  OutDataTypeStr=boolean
  Constant : Constant  OutDataTypeStr=uint32
  Delay : Delay
  Delay1 : Delay  DelayLength=1
  Delay36 : Delay  DelayLength=1
  Logical Operator : Logic  Operator=NOT  AllPortsSameDT=off  OutDataTypeStr=boolean
  Logical Operator1 : Logic  Operator=OR  AllPortsSameDT=off  OutDataTypeStr=boolean
  Logical Operator2 : Logic  AllPortsSameDT=off  OutDataTypeStr=boolean
  Relational Operator : RelationalOperator  OutDataTypeStr=boolean  RndMeth=Nearest
  Selector1 : Selector  InputPortWidth=2  IndexOptions=Index vector (dialog)  Indices=[1]  OutputSizes=1
  Selector2 : Selector  InputPortWidth=2  IndexOptions=Index vector (dialog)  Indices=[2]  OutputSizes=1
  Selector3 : Selector  InputPortWidth=2  IndexOptions=Index vector (dialog)  Indices=[1]  OutputSizes=1
  Selector4 : Selector  InputPortWidth=2  IndexOptions=Index vector (dialog)  Indices=[2]  OutputSizes=1
  Step Counter : hdlsllib/Sources/HDL Counter  CountType=Free running  CountInit=0  CountStep=1  CountMax=2^15  CountFromType=Initial value  CountFrom=0  CountResetPort=on  CountLoadPort=off  CountEnbPort=on  CountDirPort=off  CountDataType=Unsigned  CountWordLen=32  CountFracLen=0  CountSampTime=1
  Out1 : Outport
  Out2 : Outport  Port=2
  Out3 : Outport  Port=3
  Out4 : Outport  Port=4
  Valid : Outport  Port=5
  wires:
  Selector2/1 -> Out2/1
  Delay/1 -> Selector4/1, Selector3/1
  Selector3/1 -> Out3/1
  Selector1/1 -> Out1/1
  Selector4/1 -> Out4/1
  pixel/1 -> Delay36/1, Delay/1
  Step Counter/1 -> Compare To Zero/1, Relational Operator/1
  Delay1/1 -> Logical Operator2/2, Step Counter/2, Logical Operator/1
  Logical Operator/1 -> Logical Operator1/2
  step/1 -> Add/1
  Constant/1 -> Add/2
  Add/1 -> Relational Operator/2
  Relational Operator/1 -> Logical Operator1/1
  Logical Operator1/1 -> Step Counter/1
  Compare To Zero/1 -> Logical Operator2/1
  Logical Operator2/1 -> Valid/1
  Delay36/1 -> Selector2/1, Selector1/1
  valid/1 -> Delay1/1

== system external_memory_test/DUT/2DConvPE V1.2/Address Logic/  ==
  In1 : Inport
  In2 : Inport  Port=2
  Constant1 : Constant  Value=0  OutDataTypeStr=uint32
  Constant2 : Constant  Value=0  OutDataTypeStr=uint32
  Logical Operator3 : Logic  Operator=NOT  AllPortsSameDT=off  OutDataTypeStr=boolean
  Switch : Switch  Criteria=u2 ~= 0
  Switch1 : Switch  Criteria=u2 ~= 0
  addr_bit_sel1 : hdlsllib/Logic and Bit Operations/Bit Slice  lidx=12  ridx=0
  addr_bit_sel2 : hdlsllib/Logic and Bit Operations/Bit Slice  lidx=12  ridx=0
  W : Outport
  R : Outport  Port=2
  wires:
  In2/1 -> Switch/2, Logical Operator3/1
  Constant1/1 -> Switch/1
  Switch1/1 -> addr_bit_sel1/1
  In1/1 -> Switch1/3, Switch/3
  Logical Operator3/1 -> Switch1/2
  Constant2/1 -> Switch1/1
  Switch/1 -> addr_bit_sel2/1
  addr_bit_sel1/1 -> W/1  "vec_wr_addr"
  addr_bit_sel2/1 -> R/1  "vec_wr_addr"

== system external_memory_test/DUT/2DConvPE V1.2/LIne Buffer/Line Buffer ==
  Stream_In : Inport
  Stream_Valid : Inport  Port=2
  Feature_Area : Inport  Port=3
  Feature_Width : Inport  Port=4
  CtrlGen : Subsystem
  Line Buffer : visionhdlutilities/Line Buffer  NeighborhoodSize=[3 1]  PaddingMethod=Constant  PaddingValue=0  LineBufferSize=128  SimulateUsing=Code generation
      settings: SourceProductBaseCode=VT
  pixel : Outport
  ctrl : Outport  Port=2
  shftEnable : Outport  Port=3
  wires:
  Feature_Area/1 -> CtrlGen/3(Feature_Area)
  Line Buffer/2 -> ctrl/1
  CtrlGen/1(StreamOut) -> Line Buffer/1
  Feature_Width/1 -> CtrlGen/4(Feature_Width)
  Stream_In/1 -> CtrlGen/1(Stream_In)
  CtrlGen/2(Ctrl) -> Line Buffer/2
  Stream_Valid/1 -> CtrlGen/2(Stream_Valid)
  Line Buffer/3 -> shftEnable/1
  Line Buffer/1 -> pixel/1

== system external_memory_test/DUT/2DConvPE V1.2/LIne Buffer/OutValidGen ==
  In1 : Inport
  Weight_Width : Inport  Port=2
  Feature_Height : Inport  Port=3
  Compare To Constant : simulink/Logic and Bit Operations/Compare To Constant  relop=>  const=0  OutDataTypeStr=boolean
  Constant : Constant  OutDataTypeStr=uint32  SampleTime=-1
  Delay2 : Delay  DelayLength=1
  Logical Operator1 : Logic  Operator=NOT  AllPortsSameDT=off  OutDataTypeStr=boolean
  Logical Operator2 : Logic  Operator=OR  AllPortsSameDT=off  OutDataTypeStr=boolean
  Logical Operator3 : Logic  Inputs=4  AllPortsSameDT=off  OutDataTypeStr=boolean
  Logical Operator4 : Logic  Operator=NOT  AllPortsSameDT=off  OutDataTypeStr=boolean
  Logical Operator5 : Logic  Operator=OR  AllPortsSameDT=off  OutDataTypeStr=boolean
  Logical Operator6 : Logic  Operator=NOT  Inputs=3  AllPortsSameDT=off  OutDataTypeStr=boolean
  Minus1 : Sum  Inputs=+--
  Minus2 : Sum  Inputs=+-
  NumRow_Counter : hdlsllib/Sources/HDL Counter  CountType=Free running  CountInit=0  CountStep=1  CountMax=2^15  CountFromType=Initial value  CountFrom=0  CountResetPort=on  CountLoadPort=off  CountEnbPort=on  CountDirPort=off  CountDataType=Unsigned  CountWordLen=32  CountFracLen=0  CountSampTime=1
  Pixel Control Bus Selector : BusSelector  OutputSignals=hStart,hEnd,vStart,vEnd,valid
  Relational Operator1 : RelationalOperator  Operator=<  OutDataTypeStr=boolean  RndMeth=Nearest
  Relational Operator2 : RelationalOperator  Operator=<=  OutDataTypeStr=boolean  RndMeth=Nearest
  Row_Counter : hdlsllib/Sources/HDL Counter  CountType=Free running  CountInit=0  CountStep=1  CountMax=2^15  CountFromType=Initial value  CountFrom=0  CountResetPort=on  CountLoadPort=off  CountEnbPort=on  CountDirPort=off  CountDataType=Unsigned  CountWordLen=32  CountFracLen=0  CountSampTime=1
  Terminator1 : Terminator
  valid : Outport
  wires:
  Compare To Constant/1 -> Logical Operator3/2
  NumRow_Counter/1 -> Relational Operator2/2, Compare To Constant/1
  Pixel Control Bus Selector/1 -> NumRow_Counter/2, Logical Operator2/1  "<hStart>"
  Minus2/1 -> Relational Operator2/1
  Relational Operator1/1 -> Logical Operator4/1
  Logical Operator1/1 -> Logical Operator2/2
  Pixel Control Bus Selector/3 -> Logical Operator5/1  "<vStart>"
  Feature_Height/1 -> Minus2/1
  Minus1/1 -> Relational Operator1/2
  Row_Counter/1 -> Relational Operator1/1
  Pixel Control Bus Selector/5 -> Logical Operator1/1, Row_Counter/2, Logical Operator3/3  "<valid>"
  Weight_Width/1 -> Minus1/1
  Pixel Control Bus Selector/2 -> Terminator1/1  "<hEnd>"
  Delay2/1 -> Pixel Control Bus Selector/1
  Constant/1 -> Minus1/3, Minus1/2, Minus2/2
  Logical Operator6/1 -> Logical Operator3/1
  Logical Operator5/1 -> NumRow_Counter/1
  Pixel Control Bus Selector/4 -> Logical Operator5/2  "<vEnd>"
  Relational Operator2/1 -> Logical Operator6/1
  Logical Operator2/1 -> Row_Counter/1
  Logical Operator4/1 -> Logical Operator3/4
  Logical Operator3/1 -> valid/1
  In1/1 -> Delay2/1

== system external_memory_test/DUT/2DConvPE V1.2/MaxPooling/Comparator ==
  In1 : Inport
  In2 : Inport  Port=2
  In3 : Inport  Port=3
  In4 : Inport  Port=4
  Valid : Inport  Port=5
  Delay{,1..4} (5 alike) : Delay  DelayLength=1
  Relational Operator : RelationalOperator  Operator=>  OutDataTypeStr=boolean  RndMeth=Nearest
  Relational Operator1 : RelationalOperator  Operator=>  OutDataTypeStr=boolean  RndMeth=Nearest
  Relational Operator2 : RelationalOperator  Operator=>  OutDataTypeStr=boolean  RndMeth=Nearest
  Switch : Switch  Criteria=u2 > Threshold
  Switch1 : Switch  Criteria=u2 > Threshold
  Switch2 : Switch  Criteria=u2 > Threshold
  Out1 : Outport
  outvalid : Outport  Port=2
  wires:
  Switch1/1 -> Relational Operator2/2, Switch2/3
  Switch/1 -> Switch2/1, Relational Operator2/1
  Delay/1 -> Switch/1, Relational Operator/1
  Relational Operator/1 -> Switch/2
  Relational Operator1/1 -> Switch1/2
  In2/1 -> Delay1/1
  In3/1 -> Delay2/1
  Relational Operator2/1 -> Switch2/2
  In4/1 -> Delay3/1
  Switch2/1 -> Out1/1
  Valid/1 -> Delay4/1
  Delay1/1 -> Relational Operator/2, Switch/3
  Delay2/1 -> Switch1/1, Relational Operator1/1
  In1/1 -> Delay/1
  Delay3/1 -> Relational Operator1/2, Switch1/3
  Delay4/1 -> outvalid/1

== system external_memory_test/DUT/2DConvPE V1.2/MaxPooling/Line Buffer1 ==
  Stream_In : Inport
  Stream_Valid : Inport  Port=2
  Feature_Area : Inport  Port=3
  Feature_Width : Inport  Port=4
  CtrlGen : Subsystem
  Line Buffer : visionhdlutilities/Line Buffer  NeighborhoodSize=[2 1]  PaddingMethod=Constant  PaddingValue=0  LineBufferSize=128  SimulateUsing=Code generation
      settings: SourceProductBaseCode=VT
  pixel : Outport
  ctrl : Outport  Port=2
  shftEnable : Outport  Port=3
  wires:
  Feature_Area/1 -> CtrlGen/3(Feature_Area)
  Line Buffer/2 -> ctrl/1
  CtrlGen/1(StreamOut) -> Line Buffer/1
  Feature_Width/1 -> CtrlGen/4(Feature_Width)
  Stream_In/1 -> CtrlGen/1(Stream_In)
  CtrlGen/2(Ctrl) -> Line Buffer/2
  Stream_Valid/1 -> CtrlGen/2(Stream_Valid)
  Line Buffer/3 -> shftEnable/1
  Line Buffer/1 -> pixel/1

== system external_memory_test/DUT/2DConvPE V1.2/MaxPooling/OutValidGen ==
  ctrl : Inport
  Window_Width : Inport  Port=2
  Feature_Height : Inport  Port=3
  Compare To Constant : simulink/Logic and Bit Operations/Compare To Constant  Commented=on  relop=>  const=0  OutDataTypeStr=boolean
  Constant : Constant  OutDataTypeStr=uint32  SampleTime=-1
  Delay36 : Delay  DelayLength=1
  Logical Operator1 : Logic  Operator=NOT  AllPortsSameDT=off  OutDataTypeStr=boolean
  Logical Operator3 : Logic  Inputs=3  AllPortsSameDT=off  OutDataTypeStr=boolean
  Logical Operator4 : Logic  Operator=NOT  AllPortsSameDT=off  OutDataTypeStr=boolean
  Logical Operator5 : Logic  Operator=OR  AllPortsSameDT=off  OutDataTypeStr=boolean
  Logical Operator6 : Logic  Operator=NOT  Inputs=3  AllPortsSameDT=off  OutDataTypeStr=boolean
  Minus1 : Sum  Inputs=+-
  Minus2 : Sum  Inputs=+-
  NumRow_Counter : hdlsllib/Sources/HDL Counter  CountType=Free running  CountInit=0  CountStep=1  CountMax=2^15  CountFromType=Initial value  CountFrom=0  CountResetPort=on  CountLoadPort=off  CountEnbPort=on  CountDirPort=off  CountDataType=Unsigned  CountWordLen=32  CountFracLen=0  CountSampTime=1
  Pixel Control Bus Selector : BusSelector  OutputSignals=hStart,hEnd,vStart,vEnd,valid
  Relational Operator1 : RelationalOperator  Operator=<  OutDataTypeStr=boolean  RndMeth=Nearest
  Relational Operator2 : RelationalOperator  Operator=<=  OutDataTypeStr=boolean  RndMeth=Nearest
  Row_Counter : hdlsllib/Sources/HDL Counter  CountType=Free running  CountInit=0  CountStep=1  CountMax=2^15  CountFromType=Initial value  CountFrom=0  CountResetPort=on  CountLoadPort=off  CountEnbPort=on  CountDirPort=off  CountDataType=Unsigned  CountWordLen=32  CountFracLen=0  CountSampTime=1
  Terminator1 : Terminator
  Out1 : Outport
  wires:
  NumRow_Counter/1 -> Relational Operator2/2, Compare To Constant/1
  Pixel Control Bus Selector/1 -> NumRow_Counter/2  "<hStart>"
  Minus2/1 -> Relational Operator2/1
  Relational Operator1/1 -> Logical Operator4/1
  Pixel Control Bus Selector/3 -> Logical Operator5/1  "<vStart>"
  Feature_Height/1 -> Minus2/1
  Minus1/1 -> Relational Operator1/2
  Row_Counter/1 -> Relational Operator1/1
  Pixel Control Bus Selector/5 -> Row_Counter/2, Logical Operator1/1, Logical Operator3/2  "<valid>"
  Window_Width/1 -> Minus1/1
  Pixel Control Bus Selector/2 -> Terminator1/1  "<hEnd>"
  Delay36/1 -> Pixel Control Bus Selector/1
  Constant/1 -> Minus1/2, Minus2/2
  Logical Operator6/1 -> Logical Operator3/1
  Logical Operator5/1 -> NumRow_Counter/1
  Pixel Control Bus Selector/4 -> Logical Operator5/2  "<vEnd>"
  Relational Operator2/1 -> Logical Operator6/1
  Logical Operator1/1 -> Row_Counter/1
  Logical Operator4/1 -> Logical Operator3/3
  Logical Operator3/1 -> Out1/1
  ctrl/1 -> Delay36/1

== system external_memory_test/DUT/2DConvPE V1.2/MaxPooling/window Selector ==
  pixel : Inport
  valid : Inport  Port=2
  step : Inport  Port=3
  Add : Sum  Inputs=+-
  Compare To Zero : simulink/Logic and Bit Operations/Compare To Zero  relop===  OutDataTypeStr=boolean
  Constant : Constant  OutDataTypeStr=uint32
  Delay : Delay
  Delay1 : Delay  DelayLength=1
  Delay36 : Delay  DelayLength=1
  Logical Operator : Logic  Operator=NOT  AllPortsSameDT=off  OutDataTypeStr=boolean
  Logical Operator1 : Logic  Operator=OR  AllPortsSameDT=off  OutDataTypeStr=boolean
  Logical Operator2 : Logic  AllPortsSameDT=off  OutDataTypeStr=boolean
  Relational Operator : RelationalOperator  OutDataTypeStr=boolean  RndMeth=Nearest
  Selector1 : Selector  InputPortWidth=2  IndexOptions=Index vector (dialog)  Indices=[1]  OutputSizes=1
  Selector2 : Selector  InputPortWidth=2  IndexOptions=Index vector (dialog)  Indices=[2]  OutputSizes=1
  Selector3 : Selector  InputPortWidth=2  IndexOptions=Index vector (dialog)  Indices=[1]  OutputSizes=1
  Selector4 : Selector  InputPortWidth=2  IndexOptions=Index vector (dialog)  Indices=[2]  OutputSizes=1
  Step Counter : hdlsllib/Sources/HDL Counter  CountType=Free running  CountInit=0  CountStep=1  CountMax=2^15  CountFromType=Initial value  CountFrom=0  CountResetPort=on  CountLoadPort=off  CountEnbPort=on  CountDirPort=off  CountDataType=Unsigned  CountWordLen=32  CountFracLen=0  CountSampTime=1
  Out1 : Outport
  Out2 : Outport  Port=2
  Out3 : Outport  Port=3
  Out4 : Outport  Port=4
  Valid : Outport  Port=5
  wires:
  Selector2/1 -> Out2/1
  Delay/1 -> Selector4/1, Selector3/1
  Selector3/1 -> Out3/1
  Selector1/1 -> Out1/1
  Selector4/1 -> Out4/1
  pixel/1 -> Delay36/1, Delay/1
  Step Counter/1 -> Compare To Zero/1, Relational Operator/1
  Delay1/1 -> Logical Operator2/2, Step Counter/2, Logical Operator/1
  Logical Operator/1 -> Logical Operator1/2
  step/1 -> Add/1
  Constant/1 -> Add/2
  Add/1 -> Relational Operator/2
  Relational Operator/1 -> Logical Operator1/1
  Logical Operator1/1 -> Step Counter/1
  Compare To Zero/1 -> Logical Operator2/1
  Logical Operator2/1 -> Valid/1
  Delay36/1 -> Selector2/1, Selector1/1
  valid/1 -> Delay1/1
